simulink model "FSAC2021_V1"  (R2014a)
settings: Solver=FixedStepDiscrete  StartTime=0.0  StopTime=inf  FixedStep=0.0005  RelTol=1e-3
model workspace (MAT data in the model file):
  MCOS : class17 (value not decoded)
  MCOS : class17 (value not decoded)
  MCOS : class17 (value not decoded)
  MCOS : class17 (value not decoded)
  MCOS : class17 (value not decoded)
  MCOS : class17 (value not decoded)
  MCOS : class17 (value not decoded)
  MCOS : class17 (value not decoded)
  MCOS : class17 (value not decoded)
  MCOS : class17 (value not decoded)
  MCOS : class17 (value not decoded)
  MCOS : class17 (value not decoded)
  MCOS : class17 (value not decoded)
  MCOS : class17 (value not decoded)
  MCOS : class17 (value not decoded)
  MCOS : class17 (value not decoded)
  MCOS : class17 (value not decoded)
  MCOS : class17 (value not decoded)
  MCOS : class17 (value not decoded)
  BUZZER_START = 1
  MCOS : class17 (value not decoded)
  MCOS : class17 (value not decoded)
  MCOS : class17 (value not decoded)
  MCOS : class17 (value not decoded)
  MCOS : class17 (value not decoded)
  MCOS : class17 (value not decoded)
  MCOS : class17 (value not decoded)
  MCOS : class17 (value not decoded)
  MCOS : class17 (value not decoded)
  MCOS : class17 (value not decoded)
  MCOS : class17 (value not decoded)
  MCOS : class17 (value not decoded)
  MCOS : class17 (value not decoded)
  MCOS : class17 (value not decoded)
  MCOS : class17 (value not decoded)
  MCOS : class17 (value not decoded)
  MCOS : class17 (value not decoded)
  MCOS : class17 (value not decoded)
  MCOS : class17 (value not decoded)
  MCOS : class17 (value not decoded)
  MCOS : class17 (value not decoded)
  MCOS : class17 (value not decoded)
  MCOS : class17 (value not decoded)
  MCOS : class17 (value not decoded)
  MCOS : class17 (value not decoded)
  MCOS : class17 (value not decoded)
  MCOS : class17 (value not decoded)
  MCOS : class17 (value not decoded)
  MCOS : class17 (value not decoded)
  MCOS : class17 (value not decoded)
  MCOS : class17 (value not decoded)
  MCOS : class17 (value not decoded)
  MCOS : class17 (value not decoded)
  MCOS : class17 (value not decoded)
  MCOS : class17 (value not decoded)
  MCOS : class17 (value not decoded)
  MCOS : class17 (value not decoded)
  MCOS : class17 (value not decoded)
  Brake = 11
  MCOS : class17 (value not decoded)
  MCOS : class17 (value not decoded)
  MCOS : class17 (value not decoded)
  MCOS : class17 (value not decoded)
  MCOS : class17 (value not decoded)
  MCOS : class17 (value not decoded)
  MCOS : class17 (value not decoded)
  MCOS : class17 (value not decoded)
  Sensor_Acc_b = 101.85
  Sensor_Acc_k = -0.0185
  Str_Sen_Orig_Angle = -341
  MCOS : class17 (value not decoded)
  Tire_D = 0.47
  T = 0.05
libraries: simulink x189, ec55xxlib x135
(part 4 of 9)

== system FSAC2021_V1/Input_Process/KL_Sig_Process/Analog_Signal_Process ==
  note: 0-1500r
  note: 0-Cabli(MPa)
  note: 0-Cabli(MPa)
  note: 0-Cabli(MPa)
  note: 0-100%
  note: 0-100%
  note: 制动压力传感器0-5V对应0-5MPa
      | 制动液压：y=0.001x
  note: EBS压力传感器：0-3.3v 对应 0-1.6Mpa
      |
      | y=0.000303x
  note: 左边传感器：O=0.045i-90
  note: 右边传感器：O=-0.042i+100.8
  Acc_Lft_Disp_mv : Inport
  Acc_Right_Disp_mv : Inport  Port=2
  Brk_Liquid_Prs_mv : Inport  Port=3
  EBS_GAS_Prs_1_mv : Inport  Port=4
  EBS_GAS_Prs_2_mv : Inport  Port=5
  Acc_Lft_Offset : Constant  Value=Acc_Lft_Offset
  Acc_Right_Offset : Constant  Value=408.33
  Add{,1,3..5} (5 alike) : Sum
  Brk_Liquid_Prs_Factor : Constant  Value=Brk_Liquid_Prs_Factor
  Brk_Liquid_Prs_Offset : Constant  Value=Brk_Liquid_Prs_Offset
  Compare To Constant : simulink/Logic and Bit Operations/Compare To Constant  relop=<=  const=100  OutDataTypeStr=boolean
  Constant : Constant  Value=Acc_Left_Factor
  Constant1 : Constant  Value=-0.08333
  Constant2 : Constant  Value=0
  Divide{,1,3..5} (5 alike) : Product  Inputs=**
  EBS_GAS_Prs_1_Factor : Constant
  EBS_GAS_Prs_2_Factor : Constant
  EBS_Prs_Offset : Constant  Value=0
  EBS_Prs_Offset1 : Constant  Value=0
  Gain : Gain  Gain=15
  Saturation : Saturate  UpperLimit=100  LowerLimit=0
  Saturation1 : Saturate  UpperLimit=100  LowerLimit=0
  Saturation2 : Saturate  UpperLimit=1500  LowerLimit=0
  Switch : Switch  Criteria=u2 > Threshold
  Acc_Lft_Disp_Val : Outport
  Acc_Right_Disp_Val : Outport  Port=2
  Brk_Liquid_Prs_Val : Outport  Port=3
  EBS_GAS_Prs_1_Val : Outport  Port=4
  EBS_GAS_Prs_2_Val : Outport  Port=5
  ACC : Outport  Port=6
  wires:
  Saturation/1 -> Acc_Lft_Disp_Val/1
  Add3/1 -> Brk_Liquid_Prs_Val/1
  Add4/1 -> EBS_GAS_Prs_1_Val/1
  Add5/1 -> EBS_GAS_Prs_2_Val/1
  Acc_Right_Offset/1 -> Add1/2
  Constant1/1 -> Divide1/2
  Acc_Lft_Offset/1 -> Add/2
  Divide5/1 -> Add5/1
  EBS_Prs_Offset/1 -> Add5/2
  EBS_GAS_Prs_2_Factor/1 -> Divide5/2
  EBS_GAS_Prs_2_mv/1 -> Divide5/1
  Divide3/1 -> Add3/1
  Divide4/1 -> Add4/1
  EBS_Prs_Offset1/1 -> Add4/2
  EBS_GAS_Prs_1_Factor/1 -> Divide4/2
  EBS_GAS_Prs_1_mv/1 -> Divide4/1
  Brk_Liquid_Prs_Offset/1 -> Add3/2
  Brk_Liquid_Prs_mv/1 -> Divide3/1
  Add1/1 -> Saturation1/1
  Divide1/1 -> Add1/1
  Brk_Liquid_Prs_Factor/1 -> Divide3/2
  Divide/1 -> Add/1
  Add/1 -> Saturation/1
  Constant/1 -> Divide/2
  Acc_Lft_Disp_mv/1 -> Divide/1
  Gain/1 -> Saturation2/1
  Saturation2/1 -> Acc_Right_Disp_Val/1
  Saturation1/1 -> Switch/3
  Constant2/1 -> Switch/1
  Switch/1 -> ACC/1, Gain/1
  Acc_Right_Disp_mv/1 -> Compare To Constant/1, Divide1/1
  Compare To Constant/1 -> Switch/2

== system FSAC2021_V1/Input_Process/KL_Sig_Process/Whl_Spd_Process ==
  FL_WhlSpd_Hz : Inport
  FR_WhlSpd_Hz : Inport  Port=2
  RL_WhlSpd_Hz : Inport  Port=3
  RR_WhlSpd_Hz : Inport  Port=4
  LPF : Subsystem  TreatAsAtomicUnit=on
  LPF1 : Subsystem  TreatAsAtomicUnit=on
  LPF2 : Subsystem  TreatAsAtomicUnit=on
  LPF3 : Subsystem  TreatAsAtomicUnit=on
  MeaModule : ec55xxlib/RapidECU_U2/11Calibration/MeaModule  signal=Vel_spd
  Whl2Veh_Spd_Trans : Subsystem
  Whl_Spd_Hz2RPM : Subsystem  TreatAsAtomicUnit=on
  Whl_Spd_Hz2RPM1 : Subsystem  TreatAsAtomicUnit=on
  Whl_Spd_Hz2RPM2 : Subsystem  TreatAsAtomicUnit=on
  Whl_Spd_Hz2RPM3 : Subsystem  TreatAsAtomicUnit=on
  Vel_Spd : Outport
  Whl_Spd_FL_Val : Outport  Port=2
  Whl_Spd_FF_Val : Outport  Port=3
  Whl_Spd_RL_Val : Outport  Port=4
  Whl_Spd_RR_Val : Outport  Port=5
  wires:
  LPF3/1(Filtered) -> Whl2Veh_Spd_Trans/4(Wheel_speed_leftfront_wheel), Whl_Spd_RR_Val/1
  RR_WhlSpd_Hz/1 -> Whl_Spd_Hz2RPM3/1(Whl_Spd_Hz)
  RL_WhlSpd_Hz/1 -> Whl_Spd_Hz2RPM2/1(Whl_Spd_Hz)
  FR_WhlSpd_Hz/1 -> Whl_Spd_Hz2RPM1/1(Whl_Spd_Hz)
  FL_WhlSpd_Hz/1 -> Whl_Spd_Hz2RPM/1(Whl_Spd_Hz)
  Whl_Spd_Hz2RPM/1(Whl_Spd_RPM) -> LPF/1(Filter)
  LPF2/1(Filtered) -> Whl2Veh_Spd_Trans/3(Wheel_speed_leftrear_wheel), Whl_Spd_RL_Val/1
  LPF1/1(Filtered) -> Whl2Veh_Spd_Trans/2(Wheel_speed_right_front_wheel), Whl_Spd_FF_Val/1
  LPF/1(Filtered) -> Whl2Veh_Spd_Trans/1(Wheel_speed_rightrear_wheel), Whl_Spd_FL_Val/1
  Whl_Spd_Hz2RPM2/1(Whl_Spd_RPM) -> LPF2/1(Filter)
  Whl_Spd_Hz2RPM3/1(Whl_Spd_RPM) -> LPF3/1(Filter)
  Whl2Veh_Spd_Trans/1(Vel_Speed) -> MeaModule/1
  Whl_Spd_Hz2RPM1/1(Whl_Spd_RPM) -> LPF1/1(Filter)
  MeaModule/1 -> Vel_Spd/1

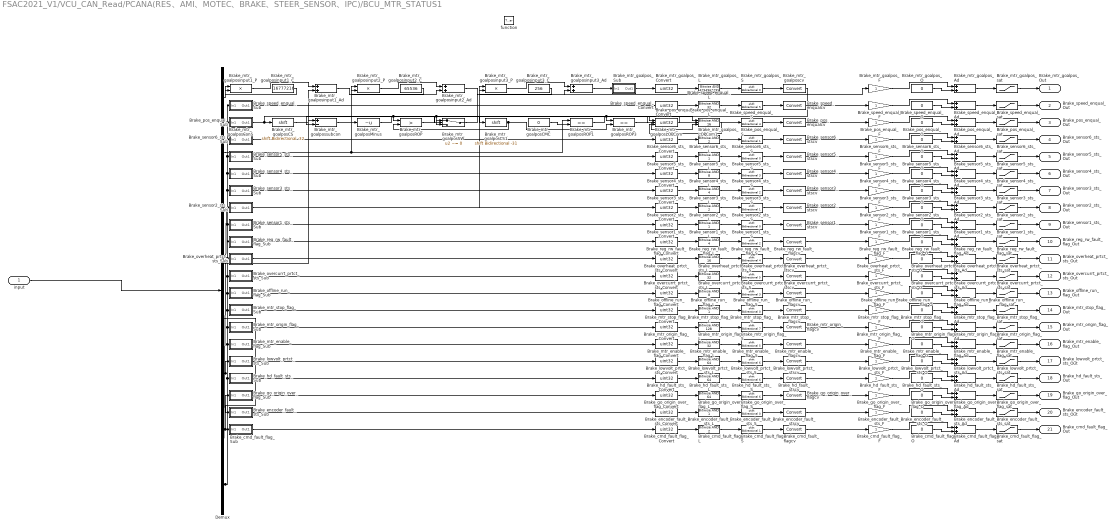
== system FSAC2021_V1/VCU_CAN_Read/PCANA(RES、AMI、MOTEC、BRAKE、STEER_SENSOR、IPC)/BCU_MTR_STATUS1 ==
  input : Inport
  function : TriggerPort  TriggerType=function-call
  Brake_cmd_fault_flag_Ad : Sum
  Brake_cmd_fault_flag_Convert : DataTypeConversion  OutDataTypeStr=uint32
  Brake_cmd_fault_flag_F : Gain
  Brake_cmd_fault_flag_L : simulink/Logic and Bit Operations/Bitwise Operator  logicop=AND  UseBitMask=on  BitMask=2  BitMaskRealWorld=Stored Integer
  Brake_cmd_fault_flag_O : Constant  Value=0  OutDataTypeStr=single
  Brake_cmd_fault_flag_S : ArithShift  BitShiftNumber=1
  Brake_cmd_fault_flag_Sub : Subsystem
  Brake_cmd_fault_flag_sat : Saturate  UpperLimit=1  LowerLimit=0
  Brake_cmd_fault_flagcv : DataTypeConversion
  Brake_encoder_fault_sts_Ad : Sum
  Brake_encoder_fault_sts_Convert : DataTypeConversion  OutDataTypeStr=uint32
  Brake_encoder_fault_sts_F : Gain
  Brake_encoder_fault_sts_L : simulink/Logic and Bit Operations/Bitwise Operator  logicop=AND  UseBitMask=on  BitMask=1  BitMaskRealWorld=Stored Integer
  Brake_encoder_fault_sts_O : Constant  Value=0  OutDataTypeStr=single
  Brake_encoder_fault_sts_S : ArithShift
  Brake_encoder_fault_sts_Sub : Subsystem
  Brake_encoder_fault_sts_sat : Saturate  UpperLimit=1  LowerLimit=0
  Brake_encoder_fault_stscv : DataTypeConversion
  Brake_go_origin_over_flag_Ad : Sum
  Brake_go_origin_over_flag_Convert : DataTypeConversion  OutDataTypeStr=uint32
  Brake_go_origin_over_flag_F : Gain
  Brake_go_origin_over_flag_L : simulink/Logic and Bit Operations/Bitwise Operator  logicop=AND  UseBitMask=on  BitMask=64  BitMaskRealWorld=Stored Integer
  Brake_go_origin_over_flag_O : Constant  Value=0  OutDataTypeStr=single
  Brake_go_origin_over_flag_S : ArithShift  BitShiftNumber=6
  Brake_go_origin_over_flag_Sub : Subsystem
  Brake_go_origin_over_flag_sat : Saturate  UpperLimit=1  LowerLimit=0
  Brake_go_origin_over_flagcv : DataTypeConversion
  Brake_hd_fault_sts_Ad : Sum
  Brake_hd_fault_sts_Convert : DataTypeConversion  OutDataTypeStr=uint32
  Brake_hd_fault_sts_F : Gain
  Brake_hd_fault_sts_L : simulink/Logic and Bit Operations/Bitwise Operator  logicop=AND  UseBitMask=on  BitMask=64  BitMaskRealWorld=Stored Integer
  Brake_hd_fault_sts_O : Constant  Value=0  OutDataTypeStr=single
  Brake_hd_fault_sts_S : ArithShift  BitShiftNumber=6
  Brake_hd_fault_sts_Sub : Subsystem
  Brake_hd_fault_sts_sat : Saturate  UpperLimit=1  LowerLimit=0
  Brake_hd_fault_stscv : DataTypeConversion
  Brake_lowvolt_prtct_sts_Ad : Sum
  Brake_lowvolt_prtct_sts_Convert : DataTypeConversion  OutDataTypeStr=uint32
  Brake_lowvolt_prtct_sts_F : Gain
  Brake_lowvolt_prtct_sts_L : simulink/Logic and Bit Operations/Bitwise Operator  logicop=AND  UseBitMask=on  BitMask=64  BitMaskRealWorld=Stored Integer
  Brake_lowvolt_prtct_sts_O : Constant  Value=0  OutDataTypeStr=single
  Brake_lowvolt_prtct_sts_S : ArithShift  BitShiftNumber=6
  Brake_lowvolt_prtct_sts_Sub : Subsystem
  Brake_lowvolt_prtct_sts_sat : Saturate  UpperLimit=1  LowerLimit=0
  Brake_lowvolt_prtct_stscv : DataTypeConversion
  Brake_mtr_enable_flag_Ad : Sum
  Brake_mtr_enable_flag_Convert : DataTypeConversion  OutDataTypeStr=uint32
  Brake_mtr_enable_flag_F : Gain
  Brake_mtr_enable_flag_L : simulink/Logic and Bit Operations/Bitwise Operator  logicop=AND  UseBitMask=on  BitMask=32  BitMaskRealWorld=Stored Integer
  Brake_mtr_enable_flag_O : Constant  Value=0  OutDataTypeStr=single
  Brake_mtr_enable_flag_S : ArithShift  BitShiftNumber=5
  Brake_mtr_enable_flag_Sub : Subsystem
  Brake_mtr_enable_flag_sat : Saturate  UpperLimit=1  LowerLimit=0
  Brake_mtr_enable_flagcv : DataTypeConversion
  Brake_mtr_goalposCMC : Constant  Value=0
  Brake_mtr_goalposCS : ArithShift  BitShiftNumber=-32
  Brake_mtr_goalposCS1 : ArithShift  BitShiftNumber=-31
  Brake_mtr_goalposConS : Constant  OutDataTypeStr=single
  Brake_mtr_goalposLOPCom : Logic  Operator=OR  AllPortsSameDT=off  OutDataTypeStr=boolean
  Brake_mtr_goalposMinus : UnaryMinus
  Brake_mtr_goalposROP : RelationalOperator  Operator=>  OutDataTypeStr=boolean
  Brake_mtr_goalposROP1 : RelationalOperator  Operator===  OutDataTypeStr=boolean
  Brake_mtr_goalposROP3 : RelationalOperator  Operator===  OutDataTypeStr=boolean
  Brake_mtr_goalposSW : Switch  Criteria=u2 ~= 0
  Brake_mtr_goalpos_Ad : Sum
  Brake_mtr_goalpos_Convert : DataTypeConversion  OutDataTypeStr=uint32
  Brake_mtr_goalpos_F : Gain
  Brake_mtr_goalpos_L : simulink/Logic and Bit Operations/Bitwise Operator  logicop=AND  UseBitMask=on  BitMask=4294967295  BitMaskRealWorld=Stored Integer
  Brake_mtr_goalpos_LOPCom1 : Logic  AllPortsSameDT=off  OutDataTypeStr=boolean
  Brake_mtr_goalpos_O : Constant  Value=0  OutDataTypeStr=single
  Brake_mtr_goalpos_S : ArithShift
  Brake_mtr_goalpos_Sub : Subsystem
  Brake_mtr_goalpos_sat : Saturate  UpperLimit=2147483647  LowerLimit=-2147483648
  Brake_mtr_goalposcv : DataTypeConversion
  Brake_mtr_goalposinput1_Ad : Sum
  Brake_mtr_goalposinput1_C : Constant  Value=16777216
  Brake_mtr_goalposinput1_P : Product
  Brake_mtr_goalposinput2_Ad : Sum
  Brake_mtr_goalposinput2_C : Constant  Value=65536
  Brake_mtr_goalposinput2_P : Product
  Brake_mtr_goalposinput3_Ad : Sum
  Brake_mtr_goalposinput3_C : Constant  Value=256
  Brake_mtr_goalposinput3_P : Product
  Brake_mtr_goalpossubcon : Sum  Inputs=+-
  Brake_mtr_origin_flag_Ad : Sum
  Brake_mtr_origin_flag_Convert : DataTypeConversion  OutDataTypeStr=uint32
  Brake_mtr_origin_flag_F : Gain
  Brake_mtr_origin_flag_L : simulink/Logic and Bit Operations/Bitwise Operator  logicop=AND  UseBitMask=on  BitMask=128  BitMaskRealWorld=Stored Integer
  Brake_mtr_origin_flag_O : Constant  Value=0  OutDataTypeStr=single
  Brake_mtr_origin_flag_S : ArithShift  BitShiftNumber=7
  Brake_mtr_origin_flag_Sub : Subsystem
  Brake_mtr_origin_flag_sat : Saturate  UpperLimit=1  LowerLimit=0
  Brake_mtr_origin_flagcv : DataTypeConversion
  Brake_mtr_stop_flag_Ad : Sum
  Brake_mtr_stop_flag_Convert : DataTypeConversion  OutDataTypeStr=uint32
  Brake_mtr_stop_flag_F : Gain
  Brake_mtr_stop_flag_L : simulink/Logic and Bit Operations/Bitwise Operator  logicop=AND  UseBitMask=on  BitMask=1  BitMaskRealWorld=Stored Integer
  Brake_mtr_stop_flag_O : Constant  Value=0  OutDataTypeStr=single
  Brake_mtr_stop_flag_S : ArithShift
  Brake_mtr_stop_flag_Sub : Subsystem
  Brake_mtr_stop_flag_sat : Saturate  UpperLimit=1  LowerLimit=0
  Brake_mtr_stop_flagcv : DataTypeConversion
  Brake_offline_run_flag_Ad : Sum
  Brake_offline_run_flag_Convert : DataTypeConversion  OutDataTypeStr=uint32
  Brake_offline_run_flag_F : Gain
  Brake_offline_run_flag_L : simulink/Logic and Bit Operations/Bitwise Operator  logicop=AND  UseBitMask=on  BitMask=8  BitMaskRealWorld=Stored Integer
  Brake_offline_run_flag_O : Constant  Value=0  OutDataTypeStr=single
  Brake_offline_run_flag_S : ArithShift  BitShiftNumber=3
  Brake_offline_run_flag_Sub : Subsystem
  Brake_offline_run_flag_sat : Saturate  UpperLimit=1  LowerLimit=0
  Brake_offline_run_flagcv : DataTypeConversion
  Brake_overcurrt_prtct_sts_Ad : Sum
  Brake_overcurrt_prtct_sts_Convert : DataTypeConversion  OutDataTypeStr=uint32
  Brake_overcurrt_prtct_sts_F : Gain
  Brake_overcurrt_prtct_sts_L : simulink/Logic and Bit Operations/Bitwise Operator  logicop=AND  UseBitMask=on  BitMask=32  BitMaskRealWorld=Stored Integer
  Brake_overcurrt_prtct_sts_O : Constant  Value=0  OutDataTypeStr=single
  Brake_overcurrt_prtct_sts_S : ArithShift  BitShiftNumber=5
  Brake_overcurrt_prtct_sts_Sub : Subsystem
  Brake_overcurrt_prtct_sts_sat : Saturate  UpperLimit=1  LowerLimit=0
  Brake_overcurrt_prtct_stscv : DataTypeConversion
  Brake_overheat_prtct_sts_Ad : Sum
  Brake_overheat_prtct_sts_Convert : DataTypeConversion  OutDataTypeStr=uint32
  Brake_overheat_prtct_sts_F : Gain
  Brake_overheat_prtct_sts_L : simulink/Logic and Bit Operations/Bitwise Operator  logicop=AND  UseBitMask=on  BitMask=16  BitMaskRealWorld=Stored Integer
  Brake_overheat_prtct_sts_O : Constant  Value=0  OutDataTypeStr=single
  Brake_overheat_prtct_sts_S : ArithShift  BitShiftNumber=4
  Brake_overheat_prtct_sts_Sub : Subsystem
  Brake_overheat_prtct_sts_sat : Saturate  UpperLimit=1  LowerLimit=0
  Brake_overheat_prtct_stscv : DataTypeConversion
  Brake_pos_enqual_Ad : Sum
  Brake_pos_enqual_Convert : DataTypeConversion  OutDataTypeStr=uint32
  Brake_pos_enqual_F : Gain
  Brake_pos_enqual_L : simulink/Logic and Bit Operations/Bitwise Operator  logicop=AND  UseBitMask=on  BitMask=16  BitMaskRealWorld=Stored Integer
  Brake_pos_enqual_O : Constant  Value=0  OutDataTypeStr=single
  Brake_pos_enqual_S : ArithShift  BitShiftNumber=4
  Brake_pos_enqual_Sub : Subsystem
  Brake_pos_enqual_sat : Saturate  UpperLimit=1  LowerLimit=0
  Brake_pos_enqualcv : DataTypeConversion
  Brake_reg_rw_fault_flag_Ad : Sum
  Brake_reg_rw_fault_flag_Convert : DataTypeConversion  OutDataTypeStr=uint32
  Brake_reg_rw_fault_flag_F : Gain
  Brake_reg_rw_fault_flag_L : simulink/Logic and Bit Operations/Bitwise Operator  logicop=AND  UseBitMask=on  BitMask=4  BitMaskRealWorld=Stored Integer
  Brake_reg_rw_fault_flag_O : Constant  Value=0  OutDataTypeStr=single
  Brake_reg_rw_fault_flag_S : ArithShift  BitShiftNumber=2
  Brake_reg_rw_fault_flag_Sub : Subsystem
  Brake_reg_rw_fault_flag_sat : Saturate  UpperLimit=1  LowerLimit=0
  Brake_reg_rw_fault_flagcv : DataTypeConversion
  Brake_sensor1_sts_Ad : Sum
  Brake_sensor1_sts_Convert : DataTypeConversion  OutDataTypeStr=uint32
  Brake_sensor1_sts_F : Gain
  Brake_sensor1_sts_L : simulink/Logic and Bit Operations/Bitwise Operator  logicop=AND  UseBitMask=on  BitMask=1  BitMaskRealWorld=Stored Integer
  Brake_sensor1_sts_O : Constant  Value=0  OutDataTypeStr=single
  Brake_sensor1_sts_S : ArithShift
  Brake_sensor1_sts_Sub : Subsystem
  Brake_sensor1_sts_sat : Saturate  UpperLimit=1  LowerLimit=0
  Brake_sensor1_stscv : DataTypeConversion
  Brake_sensor2_sts_Ad : Sum
  Brake_sensor2_sts_Convert : DataTypeConversion  OutDataTypeStr=uint32
  Brake_sensor2_sts_F : Gain
  Brake_sensor2_sts_L : simulink/Logic and Bit Operations/Bitwise Operator  logicop=AND  UseBitMask=on  BitMask=2  BitMaskRealWorld=Stored Integer
  Brake_sensor2_sts_O : Constant  Value=0  OutDataTypeStr=single
  Brake_sensor2_sts_S : ArithShift  BitShiftNumber=1
  Brake_sensor2_sts_Sub : Subsystem
  Brake_sensor2_sts_sat : Saturate  UpperLimit=1  LowerLimit=0
  Brake_sensor2_stscv : DataTypeConversion
  Brake_sensor3_sts_Ad : Sum
  Brake_sensor3_sts_Convert : DataTypeConversion  OutDataTypeStr=uint32
  Brake_sensor3_sts_F : Gain
  Brake_sensor3_sts_L : simulink/Logic and Bit Operations/Bitwise Operator  logicop=AND  UseBitMask=on  BitMask=4  BitMaskRealWorld=Stored Integer
  Brake_sensor3_sts_O : Constant  Value=0  OutDataTypeStr=single
  Brake_sensor3_sts_S : ArithShift  BitShiftNumber=2
  Brake_sensor3_sts_Sub : Subsystem
  Brake_sensor3_sts_sat : Saturate  UpperLimit=1  LowerLimit=0
  Brake_sensor3_stscv : DataTypeConversion
  Brake_sensor4_sts_Ad : Sum
  Brake_sensor4_sts_Convert : DataTypeConversion  OutDataTypeStr=uint32
  Brake_sensor4_sts_F : Gain
  Brake_sensor4_sts_L : simulink/Logic and Bit Operations/Bitwise Operator  logicop=AND  UseBitMask=on  BitMask=8  BitMaskRealWorld=Stored Integer
  Brake_sensor4_sts_O : Constant  Value=0  OutDataTypeStr=single
  Brake_sensor4_sts_S : ArithShift  BitShiftNumber=3
  Brake_sensor4_sts_Sub : Subsystem
  Brake_sensor4_sts_sat : Saturate  UpperLimit=1  LowerLimit=0
  Brake_sensor4_stscv : DataTypeConversion
  Brake_sensor5_sts_Ad : Sum
  Brake_sensor5_sts_Convert : DataTypeConversion  OutDataTypeStr=uint32
  Brake_sensor5_sts_F : Gain
  Brake_sensor5_sts_L : simulink/Logic and Bit Operations/Bitwise Operator  logicop=AND  UseBitMask=on  BitMask=1  BitMaskRealWorld=Stored Integer
  Brake_sensor5_sts_O : Constant  Value=0  OutDataTypeStr=single
  Brake_sensor5_sts_S : ArithShift
  Brake_sensor5_sts_Sub : Subsystem
  Brake_sensor5_sts_sat : Saturate  UpperLimit=1  LowerLimit=0
  Brake_sensor5_stscv : DataTypeConversion
  Brake_sensor6_sts_Ad : Sum
  Brake_sensor6_sts_Convert : DataTypeConversion  OutDataTypeStr=uint32
  Brake_sensor6_sts_F : Gain
  Brake_sensor6_sts_L : simulink/Logic and Bit Operations/Bitwise Operator  logicop=AND  UseBitMask=on  BitMask=2  BitMaskRealWorld=Stored Integer
  Brake_sensor6_sts_O : Constant  Value=0  OutDataTypeStr=single
  Brake_sensor6_sts_S : ArithShift  BitShiftNumber=1
  Brake_sensor6_sts_Sub : Subsystem
  Brake_sensor6_sts_sat : Saturate  UpperLimit=1  LowerLimit=0
  Brake_sensor6_stscv : DataTypeConversion
  Brake_speed_enqual_Ad : Sum
  Brake_speed_enqual_Convert : DataTypeConversion  OutDataTypeStr=uint32
  Brake_speed_enqual_F : Gain
  Brake_speed_enqual_L : simulink/Logic and Bit Operations/Bitwise Operator  logicop=AND  UseBitMask=on  BitMask=32  BitMaskRealWorld=Stored Integer
  Brake_speed_enqual_O : Constant  Value=0  OutDataTypeStr=single
  Brake_speed_enqual_S : ArithShift  BitShiftNumber=5
  Brake_speed_enqual_Sub : Subsystem
  Brake_speed_enqual_sat : Saturate  UpperLimit=1  LowerLimit=0
  Brake_speed_enqualcv : DataTypeConversion
  Demux : Demux  Outputs=8
  Brake_mtr_goalpos_Out : Outport
  Brake_speed_enqual_Out : Outport  Port=2
  Brake_pos_enqual_Out : Outport  Port=3
  Brake_sensor6_sts_Out : Outport  Port=4
  Brake_sensor5_sts_Out : Outport  Port=5
  Brake_sensor4_sts_Out : Outport  Port=6
  Brake_sensor3_sts_Out : Outport  Port=7
  Brake_sensor2_sts_Out : Outport  Port=8
  Brake_sensor1_sts_Out : Outport  Port=9
  Brake_reg_rw_fault_flag_Out : Outport  Port=10
  Brake_overheat_prtct_sts_Out : Outport  Port=11
  Brake_overcurrt_prtct_sts_Out : Outport  Port=12
  Brake_offline_run_flag_Out : Outport  Port=13
  Brake_mtr_stop_flag_Out : Outport  Port=14
  Brake_mtr_origin_flag_Out : Outport  Port=15
  Brake_mtr_enable_flag_Out : Outport  Port=16
  Brake_lowvolt_prtct_sts_Out : Outport  Port=17
  Brake_hd_fault_sts_Out : Outport  Port=18
  Brake_go_origin_over_flag_Out : Outport  Port=19
  Brake_encoder_fault_sts_Out : Outport  Port=20
  Brake_cmd_fault_flag_Out : Outport  Port=21
  wires:
  Brake_mtr_goalpos_F/1 -> Brake_mtr_goalpos_Ad/1
  Brake_mtr_goalpos_O/1 -> Brake_mtr_goalpos_Ad/2
  Brake_mtr_goalpos_Ad/1 -> Brake_mtr_goalpos_sat/1
  Brake_mtr_goalpos_sat/1 -> Brake_mtr_goalpos_Out/1
  Demux/1 -> Brake_mtr_goalposinput1_P/1
  Brake_mtr_goalposinput1_C/1 -> Brake_mtr_goalposinput1_P/2
  Brake_mtr_goalposinput1_P/1 -> Brake_mtr_goalposinput1_Ad/1
  Demux/4 -> Brake_mtr_goalposinput1_Ad/2
  Demux/2 -> Brake_mtr_goalposinput2_P/1, Brake_mtr_goalposROP1/1
  Brake_mtr_goalposinput2_C/1 -> Brake_mtr_goalposinput2_P/2
  Brake_mtr_goalposinput2_P/1 -> Brake_mtr_goalposinput2_Ad/1
  Brake_mtr_goalposinput1_Ad/1 -> Brake_mtr_goalposinput2_Ad/2
  Demux/3 -> Brake_mtr_goalposinput3_P/1
  Brake_mtr_goalposinput3_C/1 -> Brake_mtr_goalposinput3_P/2
  Brake_mtr_goalposinput3_P/1 -> Brake_mtr_goalposinput3_Ad/1
  Brake_mtr_goalposinput2_Ad/1 -> Brake_mtr_goalposinput3_Ad/2
  Brake_mtr_goalposinput3_Ad/1 -> Brake_mtr_goalpos_Sub/1(In1)
  Brake_mtr_goalpos_Sub/1(Out1) -> Brake_mtr_goalpos_Convert/1
  Brake_mtr_goalpos_Convert/1 -> Brake_mtr_goalpos_L/1
  Brake_mtr_goalpos_L/1 -> Brake_mtr_goalpos_S/1
  Brake_mtr_goalpos_S/1 -> Brake_mtr_goalposcv/1
  Brake_mtr_goalposcv/1 -> Brake_mtr_goalposROP/1, Brake_mtr_goalpossubcon/2, Brake_mtr_goalposSW/3, Brake_mtr_goalposROP3/1
  Brake_mtr_goalposConS/1 -> Brake_mtr_goalposCS/1, Brake_mtr_goalposCS1/1
  Brake_mtr_goalposCS1/1 -> Brake_mtr_goalposROP/2, Brake_mtr_goalposROP3/2
  Brake_mtr_goalposCS/1 -> Brake_mtr_goalpossubcon/1
  Brake_mtr_goalpossubcon/1 -> Brake_mtr_goalposMinus/1
  Brake_mtr_goalposMinus/1 -> Brake_mtr_goalposSW/1
  Brake_mtr_goalposSW/1 -> Brake_mtr_goalpos_F/1
  Brake_mtr_goalposROP1/1 -> Brake_mtr_goalpos_LOPCom1/1
  Brake_mtr_goalposROP3/1 -> Brake_mtr_goalpos_LOPCom1/2
  Brake_mtr_goalpos_LOPCom1/1 -> Brake_mtr_goalposLOPCom/2
  Brake_mtr_goalposROP/1 -> Brake_mtr_goalposLOPCom/1
  Brake_mtr_goalposLOPCom/1 -> Brake_mtr_goalposSW/2
  Brake_mtr_goalposCMC/1 -> Brake_mtr_goalposROP1/2
  Brake_speed_enqual_F/1 -> Brake_speed_enqual_Ad/1
  Brake_speed_enqual_O/1 -> Brake_speed_enqual_Ad/2
  Brake_speed_enqual_Ad/1 -> Brake_speed_enqual_sat/1
  Brake_speed_enqual_sat/1 -> Brake_speed_enqual_Out/1
  Demux/8 -> Brake_speed_enqual_Sub/1(In1), Brake_pos_enqual_Sub/1(In1), Brake_sensor4_sts_Sub/1(In1), Brake_sensor3_sts_Sub/1(In1), Brake_sensor1_sts_Sub/1(In1), Brake_mtr_origin_flag_Sub/1(In1), Brake_hd_fault_sts_Sub/1(In1), Brake_sensor2_sts_Sub/1(In1)
  Brake_speed_enqual_Sub/1(Out1) -> Brake_speed_enqual_Convert/1
  Brake_speed_enqual_Convert/1 -> Brake_speed_enqual_L/1
  Brake_speed_enqual_L/1 -> Brake_speed_enqual_S/1
  Brake_speed_enqual_S/1 -> Brake_speed_enqualcv/1
  Brake_speed_enqualcv/1 -> Brake_speed_enqual_F/1
  Brake_pos_enqual_F/1 -> Brake_pos_enqual_Ad/1
  Brake_pos_enqual_O/1 -> Brake_pos_enqual_Ad/2
  Brake_pos_enqual_Ad/1 -> Brake_pos_enqual_sat/1
  Brake_pos_enqual_sat/1 -> Brake_pos_enqual_Out/1
  Brake_pos_enqual_Sub/1(Out1) -> Brake_pos_enqual_Convert/1
  Brake_pos_enqual_Convert/1 -> Brake_pos_enqual_L/1
  Brake_pos_enqual_L/1 -> Brake_pos_enqual_S/1
  Brake_pos_enqual_S/1 -> Brake_pos_enqualcv/1
  Brake_pos_enqualcv/1 -> Brake_pos_enqual_F/1
  Brake_sensor6_sts_F/1 -> Brake_sensor6_sts_Ad/1
  Brake_sensor6_sts_O/1 -> Brake_sensor6_sts_Ad/2
  Brake_sensor6_sts_Ad/1 -> Brake_sensor6_sts_sat/1
  Brake_sensor6_sts_sat/1 -> Brake_sensor6_sts_Out/1
  Demux/6 -> Brake_sensor6_sts_Sub/1(In1), Brake_sensor5_sts_Sub/1(In1), Brake_overheat_prtct_sts_Sub/1(In1), Brake_overcurrt_prtct_sts_Sub/1(In1), Brake_lowvolt_prtct_sts_Sub/1(In1)
  Brake_sensor6_sts_Sub/1(Out1) -> Brake_sensor6_sts_Convert/1
  Brake_sensor6_sts_Convert/1 -> Brake_sensor6_sts_L/1
  Brake_sensor6_sts_L/1 -> Brake_sensor6_sts_S/1
  Brake_sensor6_sts_S/1 -> Brake_sensor6_stscv/1
  Brake_sensor6_stscv/1 -> Brake_sensor6_sts_F/1
  Brake_sensor5_sts_F/1 -> Brake_sensor5_sts_Ad/1
  Brake_sensor5_sts_O/1 -> Brake_sensor5_sts_Ad/2
  Brake_sensor5_sts_Ad/1 -> Brake_sensor5_sts_sat/1
  Brake_sensor5_sts_sat/1 -> Brake_sensor5_sts_Out/1
  Brake_sensor5_sts_Sub/1(Out1) -> Brake_sensor5_sts_Convert/1
  Brake_sensor5_sts_Convert/1 -> Brake_sensor5_sts_L/1
  Brake_sensor5_sts_L/1 -> Brake_sensor5_sts_S/1
  Brake_sensor5_sts_S/1 -> Brake_sensor5_stscv/1
  Brake_sensor5_stscv/1 -> Brake_sensor5_sts_F/1
  Brake_sensor4_sts_F/1 -> Brake_sensor4_sts_Ad/1
  Brake_sensor4_sts_O/1 -> Brake_sensor4_sts_Ad/2
  Brake_sensor4_sts_Ad/1 -> Brake_sensor4_sts_sat/1
  Brake_sensor4_sts_sat/1 -> Brake_sensor4_sts_Out/1
  Brake_sensor4_sts_Sub/1(Out1) -> Brake_sensor4_sts_Convert/1
  Brake_sensor4_sts_Convert/1 -> Brake_sensor4_sts_L/1
  Brake_sensor4_sts_L/1 -> Brake_sensor4_sts_S/1
  Brake_sensor4_sts_S/1 -> Brake_sensor4_stscv/1
  Brake_sensor4_stscv/1 -> Brake_sensor4_sts_F/1
  Brake_sensor3_sts_F/1 -> Brake_sensor3_sts_Ad/1
  Brake_sensor3_sts_O/1 -> Brake_sensor3_sts_Ad/2
  Brake_sensor3_sts_Ad/1 -> Brake_sensor3_sts_sat/1
  Brake_sensor3_sts_sat/1 -> Brake_sensor3_sts_Out/1
  Brake_sensor3_sts_Sub/1(Out1) -> Brake_sensor3_sts_Convert/1
  Brake_sensor3_sts_Convert/1 -> Brake_sensor3_sts_L/1
  Brake_sensor3_sts_L/1 -> Brake_sensor3_sts_S/1
  Brake_sensor3_sts_S/1 -> Brake_sensor3_stscv/1
  Brake_sensor3_stscv/1 -> Brake_sensor3_sts_F/1
  Brake_sensor2_sts_F/1 -> Brake_sensor2_sts_Ad/1
  Brake_sensor2_sts_O/1 -> Brake_sensor2_sts_Ad/2
  Brake_sensor2_sts_Ad/1 -> Brake_sensor2_sts_sat/1
  Brake_sensor2_sts_sat/1 -> Brake_sensor2_sts_Out/1
  Brake_sensor2_sts_Sub/1(Out1) -> Brake_sensor2_sts_Convert/1
  Brake_sensor2_sts_Convert/1 -> Brake_sensor2_sts_L/1
  Brake_sensor2_sts_L/1 -> Brake_sensor2_sts_S/1
  Brake_sensor2_sts_S/1 -> Brake_sensor2_stscv/1
  Brake_sensor2_stscv/1 -> Brake_sensor2_sts_F/1
  Brake_sensor1_sts_F/1 -> Brake_sensor1_sts_Ad/1
  Brake_sensor1_sts_O/1 -> Brake_sensor1_sts_Ad/2
  Brake_sensor1_sts_Ad/1 -> Brake_sensor1_sts_sat/1
  Brake_sensor1_sts_sat/1 -> Brake_sensor1_sts_Out/1
  Brake_sensor1_sts_Sub/1(Out1) -> Brake_sensor1_sts_Convert/1
  Brake_sensor1_sts_Convert/1 -> Brake_sensor1_sts_L/1
  Brake_sensor1_sts_L/1 -> Brake_sensor1_sts_S/1
  Brake_sensor1_sts_S/1 -> Brake_sensor1_stscv/1
  Brake_sensor1_stscv/1 -> Brake_sensor1_sts_F/1
  Brake_reg_rw_fault_flag_F/1 -> Brake_reg_rw_fault_flag_Ad/1
  Brake_reg_rw_fault_flag_O/1 -> Brake_reg_rw_fault_flag_Ad/2
  Brake_reg_rw_fault_flag_Ad/1 -> Brake_reg_rw_fault_flag_sat/1
  Brake_reg_rw_fault_flag_sat/1 -> Brake_reg_rw_fault_flag_Out/1
  Demux/7 -> Brake_reg_rw_fault_flag_Sub/1(In1), Brake_offline_run_flag_Sub/1(In1), Brake_mtr_stop_flag_Sub/1(In1), Brake_mtr_enable_flag_Sub/1(In1), Brake_go_origin_over_flag_Sub/1(In1), Brake_cmd_fault_flag_Sub/1(In1)
  Brake_reg_rw_fault_flag_Sub/1(Out1) -> Brake_reg_rw_fault_flag_Convert/1
  Brake_reg_rw_fault_flag_Convert/1 -> Brake_reg_rw_fault_flag_L/1
  Brake_reg_rw_fault_flag_L/1 -> Brake_reg_rw_fault_flag_S/1
  Brake_reg_rw_fault_flag_S/1 -> Brake_reg_rw_fault_flagcv/1
  Brake_reg_rw_fault_flagcv/1 -> Brake_reg_rw_fault_flag_F/1
  Brake_overheat_prtct_sts_F/1 -> Brake_overheat_prtct_sts_Ad/1
  Brake_overheat_prtct_sts_O/1 -> Brake_overheat_prtct_sts_Ad/2
  Brake_overheat_prtct_sts_Ad/1 -> Brake_overheat_prtct_sts_sat/1
  Brake_overheat_prtct_sts_sat/1 -> Brake_overheat_prtct_sts_Out/1
  Brake_overheat_prtct_sts_Sub/1(Out1) -> Brake_overheat_prtct_sts_Convert/1
  Brake_overheat_prtct_sts_Convert/1 -> Brake_overheat_prtct_sts_L/1
  Brake_overheat_prtct_sts_L/1 -> Brake_overheat_prtct_sts_S/1
  Brake_overheat_prtct_sts_S/1 -> Brake_overheat_prtct_stscv/1
  Brake_overheat_prtct_stscv/1 -> Brake_overheat_prtct_sts_F/1
  Brake_overcurrt_prtct_sts_F/1 -> Brake_overcurrt_prtct_sts_Ad/1
  Brake_overcurrt_prtct_sts_O/1 -> Brake_overcurrt_prtct_sts_Ad/2
  Brake_overcurrt_prtct_sts_Ad/1 -> Brake_overcurrt_prtct_sts_sat/1
  Brake_overcurrt_prtct_sts_sat/1 -> Brake_overcurrt_prtct_sts_Out/1
  Brake_overcurrt_prtct_sts_Sub/1(Out1) -> Brake_overcurrt_prtct_sts_Convert/1
  Brake_overcurrt_prtct_sts_Convert/1 -> Brake_overcurrt_prtct_sts_L/1
  Brake_overcurrt_prtct_sts_L/1 -> Brake_overcurrt_prtct_sts_S/1
  Brake_overcurrt_prtct_sts_S/1 -> Brake_overcurrt_prtct_stscv/1
  Brake_overcurrt_prtct_stscv/1 -> Brake_overcurrt_prtct_sts_F/1
  Brake_offline_run_flag_F/1 -> Brake_offline_run_flag_Ad/1
  Brake_offline_run_flag_O/1 -> Brake_offline_run_flag_Ad/2
  Brake_offline_run_flag_Ad/1 -> Brake_offline_run_flag_sat/1
  Brake_offline_run_flag_sat/1 -> Brake_offline_run_flag_Out/1
  Brake_offline_run_flag_Sub/1(Out1) -> Brake_offline_run_flag_Convert/1
  Brake_offline_run_flag_Convert/1 -> Brake_offline_run_flag_L/1
  Brake_offline_run_flag_L/1 -> Brake_offline_run_flag_S/1
  Brake_offline_run_flag_S/1 -> Brake_offline_run_flagcv/1
  Brake_offline_run_flagcv/1 -> Brake_offline_run_flag_F/1
  Brake_mtr_stop_flag_F/1 -> Brake_mtr_stop_flag_Ad/1
  Brake_mtr_stop_flag_O/1 -> Brake_mtr_stop_flag_Ad/2
  Brake_mtr_stop_flag_Ad/1 -> Brake_mtr_stop_flag_sat/1
  Brake_mtr_stop_flag_sat/1 -> Brake_mtr_stop_flag_Out/1
  Brake_mtr_stop_flag_Sub/1(Out1) -> Brake_mtr_stop_flag_Convert/1
  Brake_mtr_stop_flag_Convert/1 -> Brake_mtr_stop_flag_L/1
  Brake_mtr_stop_flag_L/1 -> Brake_mtr_stop_flag_S/1
  Brake_mtr_stop_flag_S/1 -> Brake_mtr_stop_flagcv/1
  Brake_mtr_stop_flagcv/1 -> Brake_mtr_stop_flag_F/1
  Brake_mtr_origin_flag_F/1 -> Brake_mtr_origin_flag_Ad/1
  Brake_mtr_origin_flag_O/1 -> Brake_mtr_origin_flag_Ad/2
  Brake_mtr_origin_flag_Ad/1 -> Brake_mtr_origin_flag_sat/1
  Brake_mtr_origin_flag_sat/1 -> Brake_mtr_origin_flag_Out/1
  Brake_mtr_origin_flag_Sub/1(Out1) -> Brake_mtr_origin_flag_Convert/1
  Brake_mtr_origin_flag_Convert/1 -> Brake_mtr_origin_flag_L/1
  Brake_mtr_origin_flag_L/1 -> Brake_mtr_origin_flag_S/1
  Brake_mtr_origin_flag_S/1 -> Brake_mtr_origin_flagcv/1
  Brake_mtr_origin_flagcv/1 -> Brake_mtr_origin_flag_F/1
  Brake_mtr_enable_flag_F/1 -> Brake_mtr_enable_flag_Ad/1
  Brake_mtr_enable_flag_O/1 -> Brake_mtr_enable_flag_Ad/2
  Brake_mtr_enable_flag_Ad/1 -> Brake_mtr_enable_flag_sat/1
  Brake_mtr_enable_flag_sat/1 -> Brake_mtr_enable_flag_Out/1
  Brake_mtr_enable_flag_Sub/1(Out1) -> Brake_mtr_enable_flag_Convert/1
  Brake_mtr_enable_flag_Convert/1 -> Brake_mtr_enable_flag_L/1
  Brake_mtr_enable_flag_L/1 -> Brake_mtr_enable_flag_S/1
  Brake_mtr_enable_flag_S/1 -> Brake_mtr_enable_flagcv/1
  Brake_mtr_enable_flagcv/1 -> Brake_mtr_enable_flag_F/1
  Brake_lowvolt_prtct_sts_F/1 -> Brake_lowvolt_prtct_sts_Ad/1
  Brake_lowvolt_prtct_sts_O/1 -> Brake_lowvolt_prtct_sts_Ad/2
  Brake_lowvolt_prtct_sts_Ad/1 -> Brake_lowvolt_prtct_sts_sat/1
  Brake_lowvolt_prtct_sts_sat/1 -> Brake_lowvolt_prtct_sts_Out/1
  Brake_lowvolt_prtct_sts_Sub/1(Out1) -> Brake_lowvolt_prtct_sts_Convert/1
  Brake_lowvolt_prtct_sts_Convert/1 -> Brake_lowvolt_prtct_sts_L/1
  Brake_lowvolt_prtct_sts_L/1 -> Brake_lowvolt_prtct_sts_S/1
  Brake_lowvolt_prtct_sts_S/1 -> Brake_lowvolt_prtct_stscv/1
  Brake_lowvolt_prtct_stscv/1 -> Brake_lowvolt_prtct_sts_F/1
  Brake_hd_fault_sts_F/1 -> Brake_hd_fault_sts_Ad/1
  Brake_hd_fault_sts_O/1 -> Brake_hd_fault_sts_Ad/2
  Brake_hd_fault_sts_Ad/1 -> Brake_hd_fault_sts_sat/1
  Brake_hd_fault_sts_sat/1 -> Brake_hd_fault_sts_Out/1
  Brake_hd_fault_sts_Sub/1(Out1) -> Brake_hd_fault_sts_Convert/1
  Brake_hd_fault_sts_Convert/1 -> Brake_hd_fault_sts_L/1
  Brake_hd_fault_sts_L/1 -> Brake_hd_fault_sts_S/1
  Brake_hd_fault_sts_S/1 -> Brake_hd_fault_stscv/1
  Brake_hd_fault_stscv/1 -> Brake_hd_fault_sts_F/1
  Brake_go_origin_over_flag_F/1 -> Brake_go_origin_over_flag_Ad/1
  Brake_go_origin_over_flag_O/1 -> Brake_go_origin_over_flag_Ad/2
  Brake_go_origin_over_flag_Ad/1 -> Brake_go_origin_over_flag_sat/1
  Brake_go_origin_over_flag_sat/1 -> Brake_go_origin_over_flag_Out/1
  Brake_go_origin_over_flag_Sub/1(Out1) -> Brake_go_origin_over_flag_Convert/1
  Brake_go_origin_over_flag_Convert/1 -> Brake_go_origin_over_flag_L/1
  Brake_go_origin_over_flag_L/1 -> Brake_go_origin_over_flag_S/1
  Brake_go_origin_over_flag_S/1 -> Brake_go_origin_over_flagcv/1
  Brake_go_origin_over_flagcv/1 -> Brake_go_origin_over_flag_F/1
  Brake_encoder_fault_sts_F/1 -> Brake_encoder_fault_sts_Ad/1
  Brake_encoder_fault_sts_O/1 -> Brake_encoder_fault_sts_Ad/2
  Brake_encoder_fault_sts_Ad/1 -> Brake_encoder_fault_sts_sat/1
  Brake_encoder_fault_sts_sat/1 -> Brake_encoder_fault_sts_Out/1
  Demux/5 -> Brake_encoder_fault_sts_Sub/1(In1)
  Brake_encoder_fault_sts_Sub/1(Out1) -> Brake_encoder_fault_sts_Convert/1
  Brake_encoder_fault_sts_Convert/1 -> Brake_encoder_fault_sts_L/1
  Brake_encoder_fault_sts_L/1 -> Brake_encoder_fault_sts_S/1
  Brake_encoder_fault_sts_S/1 -> Brake_encoder_fault_stscv/1
  Brake_encoder_fault_stscv/1 -> Brake_encoder_fault_sts_F/1
  Brake_cmd_fault_flag_F/1 -> Brake_cmd_fault_flag_Ad/1
  Brake_cmd_fault_flag_O/1 -> Brake_cmd_fault_flag_Ad/2
  Brake_cmd_fault_flag_Ad/1 -> Brake_cmd_fault_flag_sat/1
  Brake_cmd_fault_flag_sat/1 -> Brake_cmd_fault_flag_Out/1
  Brake_cmd_fault_flag_Sub/1(Out1) -> Brake_cmd_fault_flag_Convert/1
  Brake_cmd_fault_flag_Convert/1 -> Brake_cmd_fault_flag_L/1
  Brake_cmd_fault_flag_L/1 -> Brake_cmd_fault_flag_S/1
  Brake_cmd_fault_flag_S/1 -> Brake_cmd_fault_flagcv/1
  Brake_cmd_fault_flagcv/1 -> Brake_cmd_fault_flag_F/1
  input/1 -> Demux/1

== system FSAC2021_V1/VCU_CAN_Read/PCANA(RES、AMI、MOTEC、BRAKE、STEER_SENSOR、IPC)/IPC_CMD1 ==
  input : Inport
  function : TriggerPort  TriggerType=function-call
  Demux : Demux  Outputs=3
  IPC_Acc_Ad : Sum
  IPC_Acc_Convert : DataTypeConversion  OutDataTypeStr=uint32
  IPC_Acc_F : Gain
  IPC_Acc_L : simulink/Logic and Bit Operations/Bitwise Operator  logicop=AND  UseBitMask=on  BitMask=255  BitMaskRealWorld=Stored Integer
  IPC_Acc_O : Constant  Value=0  OutDataTypeStr=single
  IPC_Acc_S : ArithShift
  IPC_Acc_Sub : Subsystem
  IPC_Acc_sat : Saturate  UpperLimit=100  LowerLimit=0
  IPC_Acccv : DataTypeConversion
  IPC_Brk_Ad : Sum
  IPC_Brk_Convert : DataTypeConversion  OutDataTypeStr=uint32
  IPC_Brk_F : Gain
  IPC_Brk_L : simulink/Logic and Bit Operations/Bitwise Operator  logicop=AND  UseBitMask=on  BitMask=255  BitMaskRealWorld=Stored Integer
  IPC_Brk_O : Constant  Value=0  OutDataTypeStr=single
  IPC_Brk_S : ArithShift
  IPC_Brk_Sub : Subsystem
  IPC_Brk_sat : Saturate  UpperLimit=100  LowerLimit=0
  IPC_Brkcv : DataTypeConversion
  IPC_Steer_Ad : Sum
  IPC_Steer_Convert : DataTypeConversion  OutDataTypeStr=uint32
  IPC_Steer_F : Gain
  IPC_Steer_L : simulink/Logic and Bit Operations/Bitwise Operator  logicop=AND  UseBitMask=on  BitMask=255  BitMaskRealWorld=Stored Integer
  IPC_Steer_O : Constant  Value=-120  OutDataTypeStr=single
  IPC_Steer_S : ArithShift
  IPC_Steer_Sub : Subsystem
  IPC_Steer_sat : Saturate  UpperLimit=135  LowerLimit=-120
  IPC_Steercv : DataTypeConversion
  IPC_Steer_Out : Outport
  IPC_Brk_Out : Outport  Port=2
  IPC_Acc_Out : Outport  Port=3
  wires:
  IPC_Steer_F/1 -> IPC_Steer_Ad/1
  IPC_Steer_O/1 -> IPC_Steer_Ad/2
  IPC_Steer_Ad/1 -> IPC_Steer_sat/1
  IPC_Steer_sat/1 -> IPC_Steer_Out/1
  Demux/3 -> IPC_Steer_Sub/1(In1)
  IPC_Steer_Sub/1(Out1) -> IPC_Steer_Convert/1
  IPC_Steer_Convert/1 -> IPC_Steer_L/1
  IPC_Steer_L/1 -> IPC_Steer_S/1
  IPC_Steer_S/1 -> IPC_Steercv/1
  IPC_Steercv/1 -> IPC_Steer_F/1
  IPC_Brk_F/1 -> IPC_Brk_Ad/1
  IPC_Brk_O/1 -> IPC_Brk_Ad/2
  IPC_Brk_Ad/1 -> IPC_Brk_sat/1
  IPC_Brk_sat/1 -> IPC_Brk_Out/1
  Demux/2 -> IPC_Brk_Sub/1(In1)
  IPC_Brk_Sub/1(Out1) -> IPC_Brk_Convert/1
  IPC_Brk_Convert/1 -> IPC_Brk_L/1
  IPC_Brk_L/1 -> IPC_Brk_S/1
  IPC_Brk_S/1 -> IPC_Brkcv/1
  IPC_Brkcv/1 -> IPC_Brk_F/1
  IPC_Acc_F/1 -> IPC_Acc_Ad/1
  IPC_Acc_O/1 -> IPC_Acc_Ad/2
  IPC_Acc_Ad/1 -> IPC_Acc_sat/1
  IPC_Acc_sat/1 -> IPC_Acc_Out/1
  Demux/1 -> IPC_Acc_Sub/1(In1)
  IPC_Acc_Sub/1(Out1) -> IPC_Acc_Convert/1
  IPC_Acc_Convert/1 -> IPC_Acc_L/1
  IPC_Acc_L/1 -> IPC_Acc_S/1
  IPC_Acc_S/1 -> IPC_Acccv/1
  IPC_Acccv/1 -> IPC_Acc_F/1
  input/1 -> Demux/1

== system FSAC2021_V1/VCU_CAN_Read/PCANA(RES、AMI、MOTEC、BRAKE、STEER_SENSOR、IPC)/Res_Message1 ==
  input : Inport
  function : TriggerPort  TriggerType=function-call
  Demux : Demux  Outputs=1
  Res_Run_Status_Ad : Sum
  Res_Run_Status_Convert : DataTypeConversion  OutDataTypeStr=uint32
  Res_Run_Status_F : Gain
  Res_Run_Status_L : simulink/Logic and Bit Operations/Bitwise Operator  logicop=AND  UseBitMask=on  BitMask=62  BitMaskRealWorld=Stored Integer
  Res_Run_Status_O : Constant  Value=0  OutDataTypeStr=single
  Res_Run_Status_S : ArithShift  BitShiftNumber=1
  Res_Run_Status_Sub : Subsystem
  Res_Run_Status_sat : Saturate  UpperLimit=31  LowerLimit=0
  Res_Run_Statuscv : DataTypeConversion
  Res_check_Ad : Sum
  Res_check_Convert : DataTypeConversion  OutDataTypeStr=uint32
  Res_check_F : Gain
  Res_check_L : simulink/Logic and Bit Operations/Bitwise Operator  logicop=AND  UseBitMask=on  BitMask=192  BitMaskRealWorld=Stored Integer
  Res_check_O : Constant  Value=0  OutDataTypeStr=single
  Res_check_S : ArithShift  BitShiftNumber=6
  Res_check_Sub : Subsystem
  Res_check_sat : Saturate  UpperLimit=3  LowerLimit=0
  Res_checkcv : DataTypeConversion
  Safety_Relay_Ad : Sum
  Safety_Relay_Convert : DataTypeConversion  OutDataTypeStr=uint32
  Safety_Relay_F : Gain
  Safety_Relay_L : simulink/Logic and Bit Operations/Bitwise Operator  logicop=AND  UseBitMask=on  BitMask=1  BitMaskRealWorld=Stored Integer
  Safety_Relay_O : Constant  Value=0  OutDataTypeStr=single
  Safety_Relay_S : ArithShift
  Safety_Relay_Sub : Subsystem
  Safety_Relay_sat : Saturate  UpperLimit=1  LowerLimit=0
  Safety_Relaycv : DataTypeConversion
  Safety_Relay_Out : Outport
  Res_Run_Status_Out : Outport  Port=2
  Res_check_Out : Outport  Port=3
  wires:
  Safety_Relay_F/1 -> Safety_Relay_Ad/1
  Safety_Relay_O/1 -> Safety_Relay_Ad/2
  Safety_Relay_Ad/1 -> Safety_Relay_sat/1
  Safety_Relay_sat/1 -> Safety_Relay_Out/1
  Demux/1 -> Res_Run_Status_Sub/1(In1), Res_check_Sub/1(In1), Safety_Relay_Sub/1(In1)
  Safety_Relay_Sub/1(Out1) -> Safety_Relay_Convert/1
  Safety_Relay_Convert/1 -> Safety_Relay_L/1
  Safety_Relay_L/1 -> Safety_Relay_S/1
  Safety_Relay_S/1 -> Safety_Relaycv/1
  Safety_Relaycv/1 -> Safety_Relay_F/1
  Res_Run_Status_F/1 -> Res_Run_Status_Ad/1
  Res_Run_Status_O/1 -> Res_Run_Status_Ad/2
  Res_Run_Status_Ad/1 -> Res_Run_Status_sat/1
  Res_Run_Status_sat/1 -> Res_Run_Status_Out/1
  Res_Run_Status_Sub/1(Out1) -> Res_Run_Status_Convert/1
  Res_Run_Status_Convert/1 -> Res_Run_Status_L/1
  Res_Run_Status_L/1 -> Res_Run_Status_S/1
  Res_Run_Status_S/1 -> Res_Run_Statuscv/1
  Res_Run_Statuscv/1 -> Res_Run_Status_F/1
  Res_check_F/1 -> Res_check_Ad/1
  Res_check_O/1 -> Res_check_Ad/2
  Res_check_Ad/1 -> Res_check_sat/1
  Res_check_sat/1 -> Res_check_Out/1
  Res_check_Sub/1(Out1) -> Res_check_Convert/1
  Res_check_Convert/1 -> Res_check_L/1
  Res_check_L/1 -> Res_check_S/1
  Res_check_S/1 -> Res_checkcv/1
  Res_checkcv/1 -> Res_check_F/1
  input/1 -> Demux/1

== system FSAC2021_V1/VCU_CAN_Read/PCANA(RES、AMI、MOTEC、BRAKE、STEER_SENSOR、IPC)/STEER_SENSOR_INFO1 ==
  input : Inport
  function : TriggerPort  TriggerType=function-call
  Demux : Demux  Outputs=8
  Str_Sensor_Curr_AngleCS : ArithShift  BitShiftNumber=-16
  Str_Sensor_Curr_AngleCS1 : ArithShift  BitShiftNumber=-15
  Str_Sensor_Curr_AngleConS : Constant  OutDataTypeStr=single
  Str_Sensor_Curr_AngleMinus : UnaryMinus
  Str_Sensor_Curr_AngleROP : RelationalOperator  OutDataTypeStr=boolean
  Str_Sensor_Curr_AngleSW : Switch  Criteria=u2 ~= 0
  Str_Sensor_Curr_Angle_Ad : Sum
  Str_Sensor_Curr_Angle_Convert : DataTypeConversion  OutDataTypeStr=uint32
  Str_Sensor_Curr_Angle_F : Gain  Gain=0.0625
  Str_Sensor_Curr_Angle_L : simulink/Logic and Bit Operations/Bitwise Operator  logicop=AND  UseBitMask=on  BitMask=65535  BitMaskRealWorld=Stored Integer
  Str_Sensor_Curr_Angle_O : Constant  Value=0  OutDataTypeStr=single
  Str_Sensor_Curr_Angle_S : ArithShift
  Str_Sensor_Curr_Angle_Sub : Subsystem
  Str_Sensor_Curr_Angle_sat : Saturate  UpperLimit=900  LowerLimit=-900
  Str_Sensor_Curr_Anglecv : DataTypeConversion
  Str_Sensor_Curr_Angleinput2_Ad : Sum
  Str_Sensor_Curr_Angleinput2_C : Constant  Value=256
  Str_Sensor_Curr_Angleinput2_P : Product
  Str_Sensor_Curr_Anglesubcon : Sum  Inputs=+-
  Str_Sensor_Curr_Angle_Out : Outport
  wires:
  Str_Sensor_Curr_Angle_F/1 -> Str_Sensor_Curr_Angle_Ad/1
  Str_Sensor_Curr_Angle_O/1 -> Str_Sensor_Curr_Angle_Ad/2
  Str_Sensor_Curr_Angle_Ad/1 -> Str_Sensor_Curr_Angle_sat/1
  Str_Sensor_Curr_Angle_sat/1 -> Str_Sensor_Curr_Angle_Out/1
  Demux/2 -> Str_Sensor_Curr_Angleinput2_P/1
  Str_Sensor_Curr_Angleinput2_C/1 -> Str_Sensor_Curr_Angleinput2_P/2
  Str_Sensor_Curr_Angleinput2_P/1 -> Str_Sensor_Curr_Angleinput2_Ad/1
  Demux/3 -> Str_Sensor_Curr_Angleinput2_Ad/2
  Str_Sensor_Curr_Angleinput2_Ad/1 -> Str_Sensor_Curr_Angle_Sub/1(In1)
  Str_Sensor_Curr_Angle_Sub/1(Out1) -> Str_Sensor_Curr_Angle_Convert/1
  Str_Sensor_Curr_Angle_Convert/1 -> Str_Sensor_Curr_Angle_L/1
  Str_Sensor_Curr_Angle_L/1 -> Str_Sensor_Curr_Angle_S/1
  Str_Sensor_Curr_Angle_S/1 -> Str_Sensor_Curr_Anglecv/1
  Str_Sensor_Curr_Anglecv/1 -> Str_Sensor_Curr_AngleROP/1, Str_Sensor_Curr_Anglesubcon/2, Str_Sensor_Curr_AngleSW/3
  Str_Sensor_Curr_AngleConS/1 -> Str_Sensor_Curr_AngleCS/1, Str_Sensor_Curr_AngleCS1/1
  Str_Sensor_Curr_AngleCS1/1 -> Str_Sensor_Curr_AngleROP/2
  Str_Sensor_Curr_AngleCS/1 -> Str_Sensor_Curr_Anglesubcon/1
  Str_Sensor_Curr_Anglesubcon/1 -> Str_Sensor_Curr_AngleMinus/1
  Str_Sensor_Curr_AngleMinus/1 -> Str_Sensor_Curr_AngleSW/1
  Str_Sensor_Curr_AngleSW/1 -> Str_Sensor_Curr_Angle_F/1
  Str_Sensor_Curr_AngleROP/1 -> Str_Sensor_Curr_AngleSW/2
  input/1 -> Demux/1

== system FSAC2021_V1/VCU_CAN_Read/PCANA(RES、AMI、MOTEC、BRAKE、STEER_SENSOR、IPC)/Subsystem ==
  In1 : Inport
  In2 : Inport  Port=2
  In3 : Inport  Port=3
  Enable : EnablePort
  Data Type Conversion22 : DataTypeConversion
  Data Type Conversion23 : DataTypeConversion
  Data Type Conversion24 : DataTypeConversion
  Out1 : Outport
  Out2 : Outport  Port=2
  Out3 : Outport  Port=3
  wires:
  Data Type Conversion24/1 -> Out2/1
  Data Type Conversion23/1 -> Out3/1
  In1/1 -> Data Type Conversion22/1
  In2/1 -> Data Type Conversion24/1
  In3/1 -> Data Type Conversion23/1
  Data Type Conversion22/1 -> Out1/1

== system FSAC2021_V1/VCU_CAN_Read/PCANB(BMS、DRIVE_MOTOR)/AMI_DUTY ==
  input : Inport
  function : TriggerPort  TriggerType=function-call
  Demux : Demux  Outputs=1
  assi_status_Ad : Sum
  assi_status_Convert : DataTypeConversion  OutDataTypeStr=uint32
  assi_status_F : Gain
  assi_status_L : simulink/Logic and Bit Operations/Bitwise Operator  logicop=AND  UseBitMask=on  BitMask=255  BitMaskRealWorld=Stored Integer
  assi_status_O : Constant  Value=0  OutDataTypeStr=single
  assi_status_S : ArithShift
  assi_status_Sub : Subsystem
  assi_status_sat : Saturate  UpperLimit=255  LowerLimit=0
  assi_statuscv : DataTypeConversion
  assi_status_Out : Outport
  wires:
  assi_status_F/1 -> assi_status_Ad/1
  assi_status_O/1 -> assi_status_Ad/2
  assi_status_Ad/1 -> assi_status_sat/1
  assi_status_sat/1 -> assi_status_Out/1
  Demux/1 -> assi_status_Sub/1(In1)
  assi_status_Sub/1(Out1) -> assi_status_Convert/1
  assi_status_Convert/1 -> assi_status_L/1
  assi_status_L/1 -> assi_status_S/1
  assi_status_S/1 -> assi_statuscv/1
  assi_statuscv/1 -> assi_status_F/1
  input/1 -> Demux/1

== system FSAC2021_V1/VCU_CAN_Read/PCANB(BMS、DRIVE_MOTOR)/BMS_ALARM  ==
  In1 : Inport
  function : TriggerPort  TriggerType=function-call
  BMS_HCU_ALARM : Subsystem
  Data Type Conversion{38..62} (25 alike) : DataTypeConversion  OutDataTypeStr=uint8
  ALM_VCU_OFFLINE_Out : Outport
  ALM_PRECHRG_FAIL_Out : Outport  Port=2
  ALM_LEAK_OC_Out : Outport  Port=3
  ALM_HVREL_FAIL_Out : Outport  Port=4
  ALM_HALL_BREAK_Out : Outport  Port=5
  ALM_DSCH_OCT_Out : Outport  Port=6
  ALM_DSCH_OCS_Out : Outport  Port=7
  ALM_CHRG_OCT_Out : Outport  Port=8
  ALM_CHRG_OCS_Out : Outport  Port=9
  ALM_BSU_OFFLINE_Out : Outport  Port=10
  ALM_BSU_FAULT_Out : Outport  Port=11
  ALM_BMU_FAIL_Out : Outport  Port=12
  ALM_BATT_UC_Out : Outport  Port=13
  ALM_BATT_OC_Out : Outport  Port=14
  ALM_AUX_FAIL_Out : Outport  Port=15
  ALM_BATT_UV_Out : Outport  Port=16
  ALM_BATT_OV_Out : Outport  Port=17
  ALM_BATT_DT_Out : Outport  Port=18
  ALM_BATT_DV_Out : Outport  Port=19
  ALM_CELL_TBK_Out : Outport  Port=20
  ALM_CELL_IBK_Out : Outport  Port=21
  ALM_CELL_UT_Out : Outport  Port=22
  ALM_CELL_OT_Out : Outport  Port=23
  ALM_CELL_UV_Out : Outport  Port=24
  ALM_CELL_OV_Out : Outport  Port=25
  wires:
  BMS_HCU_ALARM/22(ALM_CELL_UT_Out) -> Data Type Conversion59/1
  BMS_HCU_ALARM/25(ALM_CELL_OV_Out) -> Data Type Conversion62/1
  BMS_HCU_ALARM/20(ALM_CELL_TBK_Out) -> Data Type Conversion57/1
  BMS_HCU_ALARM/14(ALM_BATT_OC_Out) -> Data Type Conversion51/1
  BMS_HCU_ALARM/24(ALM_CELL_UV_Out) -> Data Type Conversion61/1
  BMS_HCU_ALARM/21(ALM_CELL_IBK_Out) -> Data Type Conversion58/1
  BMS_HCU_ALARM/23(ALM_CELL_OT_Out) -> Data Type Conversion60/1
  BMS_HCU_ALARM/1(ALM_VCU_OFFLINE_Out) -> Data Type Conversion38/1
  BMS_HCU_ALARM/19(ALM_BATT_DV_Out) -> Data Type Conversion56/1
  BMS_HCU_ALARM/6(ALM_DSCH_OCT_Out) -> Data Type Conversion43/1
  BMS_HCU_ALARM/17(ALM_BATT_OV_Out) -> Data Type Conversion54/1
  BMS_HCU_ALARM/18(ALM_BATT_DT_Out) -> Data Type Conversion55/1
  BMS_HCU_ALARM/7(ALM_DSCH_OCS_Out) -> Data Type Conversion44/1
  BMS_HCU_ALARM/16(ALM_BATT_UV_Out) -> Data Type Conversion53/1
  BMS_HCU_ALARM/13(ALM_BATT_UC_Out) -> Data Type Conversion50/1
  BMS_HCU_ALARM/15(ALM_AUX_FAIL_Out) -> Data Type Conversion52/1
  BMS_HCU_ALARM/8(ALM_CHRG_OCT_Out) -> Data Type Conversion45/1
  Data Type Conversion38/1 -> ALM_VCU_OFFLINE_Out/1
  BMS_HCU_ALARM/5(ALM_HALL_BREAK_Out) -> Data Type Conversion42/1
  BMS_HCU_ALARM/10(ALM_BSU_OFFLINE_Out) -> Data Type Conversion47/1
  BMS_HCU_ALARM/12(ALM_BMU_FAIL_Out) -> Data Type Conversion49/1
  BMS_HCU_ALARM/2(ALM_PRECHRG_FAIL_Out) -> Data Type Conversion40/1
  BMS_HCU_ALARM/3(ALM_LEAK_OC_Out) -> Data Type Conversion39/1
  BMS_HCU_ALARM/4(ALM_HVREL_FAIL_Out) -> Data Type Conversion41/1
  BMS_HCU_ALARM/11(ALM_BSU_FAULT_Out) -> Data Type Conversion48/1
  BMS_HCU_ALARM/9(ALM_CHRG_OCS_Out) -> Data Type Conversion46/1
  Data Type Conversion47/1 -> ALM_BSU_OFFLINE_Out/1
  Data Type Conversion41/1 -> ALM_HVREL_FAIL_Out/1
  Data Type Conversion43/1 -> ALM_HALL_BREAK_Out/1
  Data Type Conversion42/1 -> ALM_DSCH_OCT_Out/1
  Data Type Conversion45/1 -> ALM_CHRG_OCT_Out/1
  Data Type Conversion40/1 -> ALM_PRECHRG_FAIL_Out/1
  Data Type Conversion39/1 -> ALM_LEAK_OC_Out/1
  Data Type Conversion46/1 -> ALM_CHRG_OCS_Out/1
  Data Type Conversion44/1 -> ALM_DSCH_OCS_Out/1
  Data Type Conversion50/1 -> ALM_BATT_UC_Out/1
  Data Type Conversion51/1 -> ALM_BATT_OC_Out/1
  Data Type Conversion53/1 -> ALM_BATT_UV_Out/1
  Data Type Conversion54/1 -> ALM_BATT_OV_Out/1
  Data Type Conversion52/1 -> ALM_AUX_FAIL_Out/1
  Data Type Conversion48/1 -> ALM_BSU_FAULT_Out/1
  Data Type Conversion55/1 -> ALM_BATT_DT_Out/1
  Data Type Conversion56/1 -> ALM_BATT_DV_Out/1
  Data Type Conversion49/1 -> ALM_BMU_FAIL_Out/1
  Data Type Conversion61/1 -> ALM_CELL_UV_Out/1
  Data Type Conversion58/1 -> ALM_CELL_IBK_Out/1
  Data Type Conversion60/1 -> ALM_CELL_OT_Out/1
  Data Type Conversion59/1 -> ALM_CELL_UT_Out/1
  Data Type Conversion62/1 -> ALM_CELL_OV_Out/1
  Data Type Conversion57/1 -> ALM_CELL_TBK_Out/1
  In1/1 -> BMS_HCU_ALARM/1(input)
